simulink model "simulation_control_LQR_WP2"  (R2023a)
settings: Solver=VariableStepAuto  StartTime=0.0  StopTime=10.0  RelTol=1e-3
values from neighbouring files (symbols this model uses):
  K = [k1 k2]    [WP2.m]    (also in parameters_for_equipollenza_WP2.m = [8109.81 179.9]; poleplacement_WP2.m = [1609.81 39.90]; poleplacement_test1_WP2.m = [739.81 53.9]; poleplacement_test2_WP2.m = [17.1 5.3])
settings Model: Creator=giova  LastModifiedBy=giova

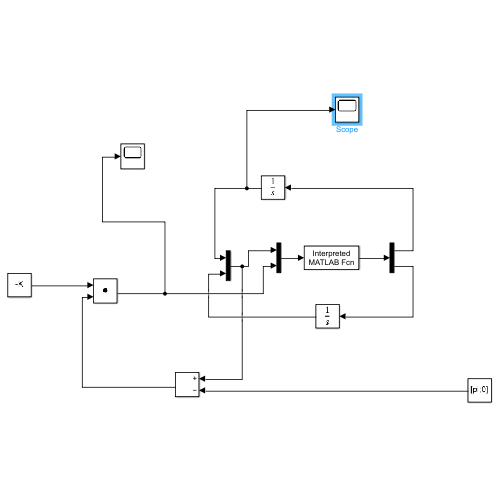
[thumbnail: Simulink's stored preview of the top-level diagram]
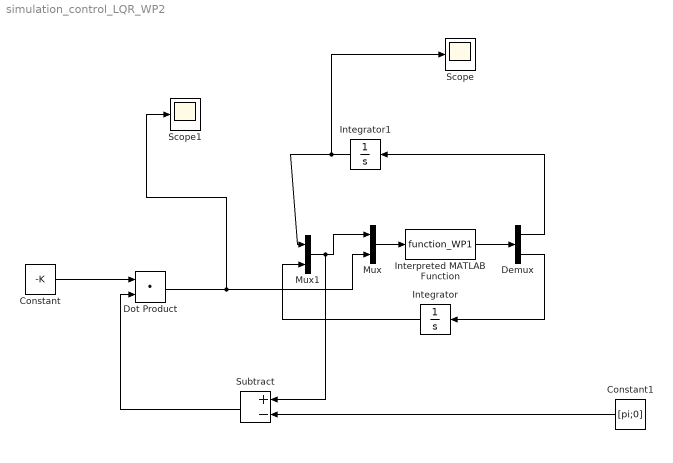
== system simulation_control_LQR_WP2 ==
  Constant : Constant  Value=-K
  Constant1 : Constant  Value=[pi;0]
  Demux : Demux  Outputs=2
  Dot Product : DotProduct  OutDataTypeStr=Inherit: Inherit via internal rule
  Integrator : Integrator
  Integrator1 : Integrator
  Interpreted MATLAB Function : MATLABFcn  MATLABFcn=function_WP1  OutputDimensions=2
  Mux : Mux  Inputs=2
  Mux1 : Mux  Inputs=2
  Scope : Scope
  Scope1 : Scope
  Subtract : Sum  Inputs=+-
  wires:
  Integrator1/1 -> Scope/1, Mux1/1
  Mux/1 -> Interpreted MATLAB Function/1
  Interpreted MATLAB Function/1 -> Demux/1
  Mux1/1 -> Subtract/1, Mux/1
  Demux/1 -> Integrator1/1
  Integrator/1 -> Mux1/2
  Demux/2 -> Integrator/1
  Constant/1 -> Dot Product/1
  Constant1/1 -> Subtract/2
  Subtract/1 -> Dot Product/2
  Dot Product/1 -> Scope1/1, Mux/2
